simulink model "controller"  (R2020a)
settings: Solver=VariableStepAuto  StartTime=0.0  StopTime=10.0  RelTol=1e-3
PostLoadFcn:
  | a = -3;
  | b = -4;
  | Kp = 36;
  | Ki = 4;
  | m = 25;
  | t = [0:0.01:10]';
  | Ts = 0.01;
  | stin = [zeros(floor((length(t)/2)+1),1) ; 5*ones(floor(length(t)/2),1)];
model workspace (MAT data in the model file):
  Var = 0
settings Model: Creator=kasutav  LastModifiedBy=kasutav
settings DataIOCC: ExternalInput=[t, stin]  LoadExternalInput=on  SaveFormat=Array  SaveOutput=off  SaveTime=off  ReturnWorkspaceOutputs=off

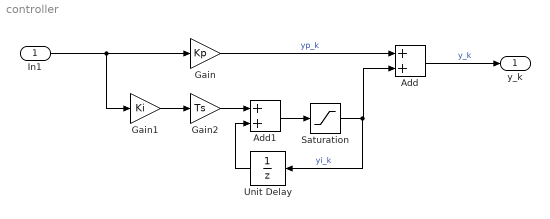
== system controller ==
  In1 : Inport  OutDataTypeStr=double  PortDimensions=1  SampleTime=0
  Add : Sum
  Add1 : Sum
  Gain : Gain  Gain=Kp
  Gain1 : Gain  Gain=Ki
  Gain2 : Gain  Gain=Ts
  Saturation : Saturate  UpperLimit=0.1  LowerLimit=-0.1
  Unit Delay : UnitDelay  SampleTime=-1  HasFrameUpgradeWarning=on
  y_k : Outport  OutDataTypeStr=double  PortDimensions=1  SampleTime=0
  wires:
  Gain2/1 -> Add1/1
  In1/1 -> Gain1/1, Gain/1
  Gain1/1 -> Gain2/1
  Unit Delay/1 -> Add1/2
  Add/1 -> y_k/1  "y_k"
  Add1/1 -> Saturation/1
  Gain/1 -> Add/1  "yp_k"
  Saturation/1 -> Add/2, Unit Delay/1  "yi_k"
